simulink model "orbitfollower3Danimation"  (R2021a)
settings: Solver=VariableStepAuto  StartTime=0.0  StopTime=10.0  RelTol=1e-3
libraries: uavalgslib x1, simulink x1, sim3dlib x1, uavsim3dlib x1
settings Model: Creator=student  LastModifiedBy=student

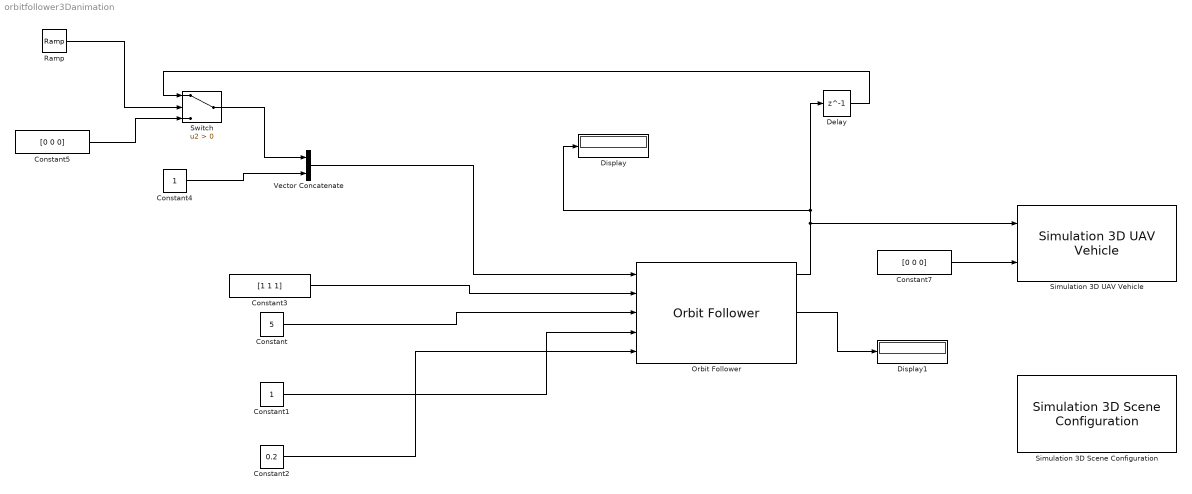
== system orbitfollower3Danimation ==
  Constant : Constant  Value=5
  Constant1 : Constant
  Constant2 : Constant  Value=0.2
  Constant3 : Constant  Value=[1 1 1]
  Constant4 : Constant
  Constant5 : Constant  Value=[0 0 0]
  Constant7 : Constant  Value=[0 0 0]
  Delay : Delay  DelayLength=1
  Display : Display
  Display1 : Display
  Orbit Follower : uavalgslib/Orbit Follower  UAVType=multirotor  MinOrbitRadius=1  MinLookaheadDistance=0.1  ExternalReset=none  ShowCrossTrackErrorOutput=off  ShowNumTurnsOutput=off  SimulateUsing=Interpreted execution
      settings: SourceProductBaseCode=UV
  Ramp : simulink/Sources/Ramp  slope=1  start=0  InitialOutput=0
  Simulation 3D Scene Configuration : sim3dlib/Simulation 3D Scene Configuration  Priority=0  ProjectFormat=Default Scenes  SceneDesc=US city block  ProjectName=C:\Program Files\MATLAB\R2021a\toolbox\shared\sim3d_projects\automotive_project\UE4\WindowsNoEditor\VehicleSimulation.exe  ScenePath=/Game/Maps/USCityBlock  vehTagList={'Scene Origin'}  vehTag=Scene Origin  OpVisEn=off  Ts=1/60  EnableWindow=on  EnableWeather=off  SunAltitude=40.0  SunAzimuth=90  clouds=10  wind=1  fog=0  rain=0  sensorTag=MainCamera1  sensorId=1  sensorName=MainCamera1  mountLoc=Origin  offsetFlag=off  tmountOffset=[0, 0, 0]  rmountOffset=[0, 0, 0]  HorizontalResolution=1280  VerticalResolution=720  HorizontalFOV=60  mountPoint=[0 0 0]  mountOrientation=[0 0 0]  aMode=4  ID=1
      settings: SourceProductBaseCode=DR,UV,VE
  Simulation 3D UAV Vehicle : uavsim3dlib/Simulation 3D UAV Vehicle  Priority=-1  Mesh=Quadrotor  Color=Black  ActorName=SimulinkVehicle1  InitialTranslation=[0 0 0]  InitialRotation=[0 0 0]  SampleTime=-1  ActorType=SimulinkVehicle  ID=1  aMode=4  ActorTag=SimulinkVehicle1
      settings: SourceProductBaseCode=UV
  Switch : Switch  Criteria=u2 > Threshold
  Vector Concatenate : Concatenate
  wires:
  Constant/1 -> Orbit Follower/3
  Constant1/1 -> Orbit Follower/4
  Constant2/1 -> Orbit Follower/5
  Constant3/1 -> Orbit Follower/2
  Constant7/1 -> Simulation 3D UAV Vehicle/2
  Constant4/1 -> Vector Concatenate/2
  Switch/1 -> Vector Concatenate/1
  Vector Concatenate/1 -> Orbit Follower/1
  Constant5/1 -> Switch/3
  Ramp/1 -> Switch/2
  Orbit Follower/3 -> Display1/1
  Delay/1 -> Switch/1
  Orbit Follower/1 -> Simulation 3D UAV Vehicle/1, Display/1, Delay/1
